simulink model "AC_motor"  (R2025b)
settings: Solver=VariableStepAuto  StartTime=0.0  StopTime=10  RelTol=1e-3
libraries: nesl_utility x11, ee_lib x10, fl_lib x8
settings Model: Creator=Администратор  LastModifiedBy=Администратор

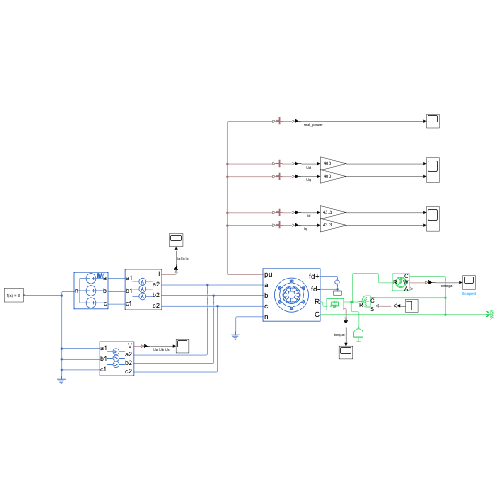
[thumbnail: Simulink's stored preview of the top-level diagram]
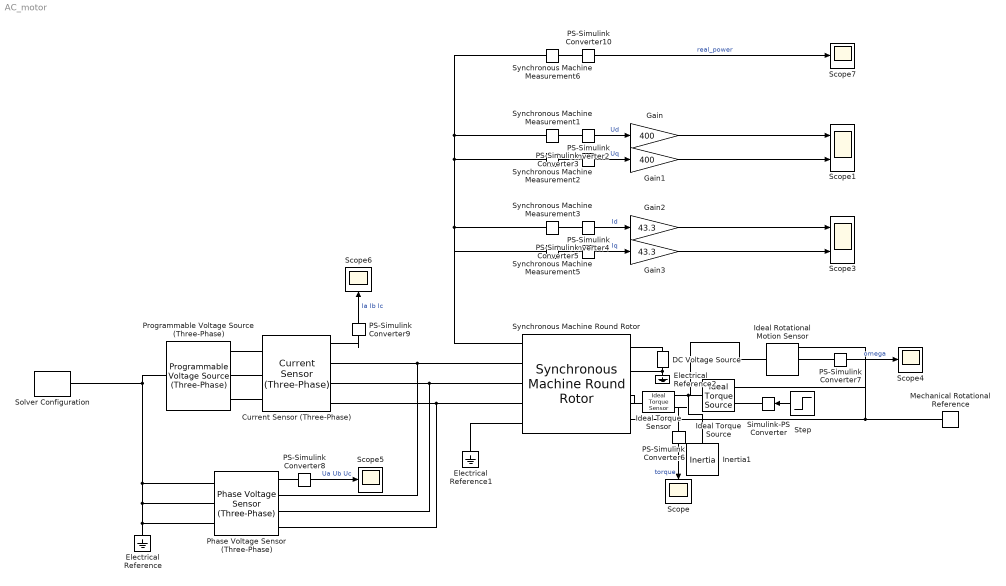
== system AC_motor ==
  Current Sensor (Three-Phase) : ee_lib/Sensors & Transducers/Current Sensor (Three-Phase)
      settings: InternalSimscapePortConfiguration="{\"Bottom\":[],\"Left\":[{\"id\":\"a1\",\"label\":\"a1\",\"type\":\"foundation.electrical.electrical\"},{\"id\":\"b1\",\"label\":\"b1\",\"type\":\"foundation.electrical.electrical\"},{\"id\":\"c1\",\"label\":\"c1\",\"type\":\"foundation.electrical.electrical\"}],\"Right\":[{\"id\":\"I_output\",\"label\":\"I\",\"type\":\"output\"},{\"id\":\"a2\",\"label\":\"a2\",\"type\":\"foundation.electrical.electrical\"},{\"id\":\"b2\",\"label\":\"b2\",\"type\":\"foundation.electrical.electrical\"},{\"id\":\"c2\",\"label\":\"c2\",\"type\":\"foundation.electrical.electrical\"}],\"Top\":[]}"
  DC Voltage Source : ee_lib/Additional Components/SPICE Sources/DC Voltage Source  DC=24 V
  Electrical Reference : fl_lib/Electrical/Electrical Elements/Electrical Reference
  Electrical Reference1 : fl_lib/Electrical/Electrical Elements/Electrical Reference
  Electrical Reference2 : fl_lib/Electrical/Electrical Elements/Electrical Reference
  Gain : Gain  Gain=400
  Gain1 : Gain  Gain=400
  Gain2 : Gain  Gain=43.3
  Gain3 : Gain  Gain=43.3
  Ideal Rotational Motion Sensor : fl_lib/Mechanical/Mechanical Sensors/Ideal Rotational Motion Sensor  reference=foundation.enum.MeasurementReference.difference  acceleration_port=false  velocity_port=true  position_port=true  wrap_angle=false  offset=0 rad
  Ideal Torque Sensor : fl_lib/Mechanical/Mechanical Sensors/Ideal Torque Sensor
  Ideal Torque Source : fl_lib/Mechanical/Mechanical Sources/Ideal Torque Source
  Inertia1 : fl_lib/Mechanical/Rotational Elements/Inertia  inertia=0.05 kg*m^2  num_ports=foundation.enum.numPorts2.one  w_specify=off  w_priority=High  w=0 rad/s  w_nominal_specify=off  w_nominal_value=1  w_nominal_unit=rad/s  t_specify=off  t_priority=None  t=0 N*m  t_nominal_specify=off  t_nominal_value=1  t_nominal_unit=N*m
  Mechanical Rotational Reference : fl_lib/Mechanical/Rotational Elements/Mechanical Rotational Reference
  PS-Simulink Converter{2..10} (9 alike) : nesl_utility/PS-Simulink Converter  PhysicalDomain=network_engine_domain  SubClassName=ps_output  LeftPortType=input  RightPortType=output  PseudoPeriodic=off  Frequencies=[]  VectorFormat=inherit  Unit=inherit  AffineConversion=off
  Phase Voltage Sensor (Three-Phase) : ee_lib/Sensors & Transducers/Phase Voltage Sensor (Three-Phase)
      settings: InternalSimscapePortConfiguration="{\"Bottom\":[],\"Left\":[{\"id\":\"a1\",\"label\":\"a1\",\"type\":\"foundation.electrical.electrical\"},{\"id\":\"b1\",\"label\":\"b1\",\"type\":\"foundation.electrical.electrical\"},{\"id\":\"c1\",\"label\":\"c1\",\"type\":\"foundation.electrical.electrical\"}],\"Right\":[{\"id\":\"V_output\",\"label\":\"V\",\"type\":\"output\"},{\"id\":\"a2\",\"label\":\"a2\",\"type\":\"foundation.electrical.electrical\"},{\"id\":\"b2\",\"label\":\"b2\",\"type\":\"foundation.electrical.electrical\"},{\"id\":\"c2\",\"label\":\"c2\",\"type\":\"foundation.electrical.electrical\"}],\"Top\":[]}"
  Programmable Voltage Source (Three-Phase) : ee_lib/Sources/Programmable Voltage Source (Three-Phase)  magnitude_type=ee.enum.timechanging.constant  vline_rms=400 V  magn_ramp=1 V/s  magn_step=1 V  magn_modu_magn=1 V  magn_modu_freq=1 Hz  magn_t1=1 s  magn_t2=2 s  frequency_type=ee.enum.timechanging.constant  freq=50 Hz  freq_ramp=1 Hz/s  freq_step=1 Hz  freq_modu_magn=1 Hz  freq_modu_freq=1 Hz  freq_t1=1 s  freq_t2=2 s  phase_type=ee.enum.timechanging.constant  shift=0 deg  phase_ramp=1 deg/s  phase_step=1 deg  phase_modu_magn=1 deg  phase_modu_freq=1 Hz  phase_t1=1 s  phase_t2=2 s  impedance_option=1  SShortCircuit=1e6 A*V  XR=15  R=0.01 Ohm  L=3.97e-4 H  G_parasitic=1e-6 1/Ohm  harmonic_option=0  harmonic_orders=[5, 7, 11, 13]  harmonic_ratios=[.1, .1, .1, .1]  harmonic_shifts=[0, 0, 0, 0] deg  harmonic_sequences=[1, 1, 1, 1]  harmonic_t1=-inf s  harmonic_t2=inf s  I_specify=off  I_priority=None  I=[0, 0, 0] A  I_nominal_specify=off  I_nominal_value=1  I_nominal_unit=A  V_specify=off  V_priority=None  V=[0, 0, 0] V  V_nominal_specify=off  V_nominal_value=1  V_nominal_unit=V
      settings: InternalSimscapePortConfiguration="{\"Bottom\":[],\"Left\":[{\"id\":\"n\",\"label\":\"n\",\"type\":\"foundation.electrical.electrical\"}],\"Right\":[{\"id\":\"a\",\"label\":\"a\",\"type\":\"foundation.electrical.electrical\"},{\"id\":\"b\",\"label\":\"b\",\"type\":\"foundation.electrical.electrical\"},{\"id\":\"c\",\"label\":\"c\",\"type\":\"foundation.electrical.electrical\"}],\"Top\":[]}"
  Scope{,4..7} (5 alike) : Scope
      Scope settings: ActiveDisplayYMinimum=-180.7119358740091  ActiveDisplayYMaximum=164.56605667800315  DataLoggingVariableName=ScopeData3
      Scope4 settings: ActiveDisplayYMinimum=121.85410021778432  ActiveDisplayYMaximum=208.87010775351609  DataLoggingVariableName=ScopeData4
      Scope5 settings: ActiveDisplayYMinimum=-4339.2016290441516  ActiveDisplayYMaximum=1807.2818447656446  DataLoggingVariableName=ScopeData5
      Scope6 settings: ActiveDisplayYMinimum=-436.89999743649622  ActiveDisplayYMaximum=142.21320753429535  DataLoggingVariableName=ScopeData6
      Scope7 settings: ActiveDisplayYMinimum=-0.70641268155042636  ActiveDisplayYMaximum=-0.5696896154734612  DataLoggingVariableName=ScopeData7
  Scope1 : Scope  NumInputPorts=2
      settings: ActiveDisplayYMinimum=-0.68803937842332719  ActiveDisplayYMaximum=0.70916847198511146
  Scope3 : Scope  NumInputPorts=2
      settings: ActiveDisplayYMinimum=-1.0232590834035449  ActiveDisplayYMaximum=0.66835925847558086
  Simulink-PS Converter : nesl_utility/Simulink-PS Converter  PhysicalDomain=network_engine_domain  SubClassName=ps_input  LeftPortType=input  RightPortType=output  PseudoPeriodic=off  Frequencies=[]  NoiseDistribution=none  NoiseParameters=[]  Unit=1  AffineConversion=off  FilteringAndDerivatives=provide  SimscapeFilterOrder=1  InputFilterTimeConstant=0.001  UdotUserProvided=0
  Solver Configuration : nesl_utility/Solver Configuration  PhysicalDomain=network_engine_domain  SubClassName=solver  LeftPortType=input  RightPortType=generic  Tones=[]  Harmonics=[]  SimulateNoise=off  Profile=off  UseLocalSampling=off  EnableSwitchedLinearOptims=on  FrequencyDomain=off  UseCCode=off  RelTol=0.001  AbsTol=0.001  MinStep=1e-09  ToWorkspace=off  RevertToSquareIcSolve=off  NumHomotopyIterations=100  PhasorMode=off  PhasorModeNumHarmonics=1  ConsistencySolver=NEWTON_XTOL_AFTER_FTOL  IndexReductionMethod=DerivativeReplacement  DoDC=off  ResidualTolerance=1e-09  ConsistencyTolSource=GLOBAL  ConsistencyAbsTol=0.001  ConsistencyRelTol=0.001  ConsistencyTolFactor=0.001  UseLocalSolver=off  LocalSolverChoice=NE_BACKWARD_EULER_ADVANCER  ResolveIndetEquations=on  FunctionEvalNumThread=1  LocalSolverSampleTime=0.001  DoFixedCost=off  MaxNonlinIter=3  MaxModeIter=2  ComputeImpulses=off  ImpulseIterations=2  LinearAlgebra=auto  LinearAlgebraNumThread=0  EquationFormulation=NE_TIME_EF  DelaysMemoryBudget=1024  AutomaticFiltering=on  FilteringTimeConstant=0.001  PartitionStorageMethod=AS_NEEDED  PartitionMemoryBudget=1024  PartitionMethod=ROBUST  MultibodyUseLocalSolver=off  MultibodyLocalSolverChoice=ODE1  MultibodyLocalSolverSampleTime=0.001
  Step : Step  Time=5  After=-100  SampleTime=0
  Synchronous Machine Measurement1 : ee_lib/Electromechanical/Synchronous/Synchronous Machine Measurement  output_idx=5
      settings: InternalSimscapePortConfiguration="{\"Bottom\":[],\"Left\":[{\"id\":\"pu_input\",\"label\":\"pu\",\"type\":\"input\"}],\"Right\":[{\"id\":\"pu_output\",\"label\":\"o\",\"type\":\"output\"}],\"Top\":[]}"
  Synchronous Machine Measurement2 : ee_lib/Electromechanical/Synchronous/Synchronous Machine Measurement  output_idx=6
      settings: InternalSimscapePortConfiguration="{\"Bottom\":[],\"Left\":[{\"id\":\"pu_input\",\"label\":\"pu\",\"type\":\"input\"}],\"Right\":[{\"id\":\"pu_output\",\"label\":\"o\",\"type\":\"output\"}],\"Top\":[]}"
  Synchronous Machine Measurement3 : ee_lib/Electromechanical/Synchronous/Synchronous Machine Measurement  output_idx=8
      settings: InternalSimscapePortConfiguration="{\"Bottom\":[],\"Left\":[{\"id\":\"pu_input\",\"label\":\"pu\",\"type\":\"input\"}],\"Right\":[{\"id\":\"pu_output\",\"label\":\"o\",\"type\":\"output\"}],\"Top\":[]}"
  Synchronous Machine Measurement5 : ee_lib/Electromechanical/Synchronous/Synchronous Machine Measurement  output_idx=9
      settings: InternalSimscapePortConfiguration="{\"Bottom\":[],\"Left\":[{\"id\":\"pu_input\",\"label\":\"pu\",\"type\":\"input\"}],\"Right\":[{\"id\":\"pu_output\",\"label\":\"o\",\"type\":\"output\"}],\"Top\":[]}"
  Synchronous Machine Measurement6 : ee_lib/Electromechanical/Synchronous/Synchronous Machine Measurement  output_idx=12
      settings: InternalSimscapePortConfiguration="{\"Bottom\":[],\"Left\":[{\"id\":\"pu_input\",\"label\":\"pu\",\"type\":\"input\"}],\"Right\":[{\"id\":\"pu_output\",\"label\":\"o\",\"type\":\"output\"}],\"Top\":[]}"
  Synchronous Machine Round Rotor : ee_lib/Electromechanical/Synchronous/Synchronous Machine Round Rotor  port_option=ee.enum.threePhasePort.expanded  SRated=30e3 A*V  VRated=400 V  FRated=50 Hz  nPolePairs=2  param_option=ee.enum.sm.parameterization.fundamental  fieldCircuitParameterization_option=ee.enum.sm.fieldparameterization.voltage  baseEfd=24 V  baseIfd=1300 A  zero_sequence=ee.enum.park.zerosequence.include  axes_param=ee.enum.rotorangle.daxis  Ladu=0.03  Laqu=0.03  L0=0.005  Ll=0.005  Ra=0.1  Lfd=0.05  Rfd=2  L1d=0.01  R1d=1  L1q=0.01  R1q=1  L2q=0.005  R2q=1  Xl=0.15  Xd=1.81  Xq=1.76  X0=0.15  Xdd=0.3  Xqd=0.65  Xddd=0.23  Xqdd=0.25  d_option=ee.enum.circuit.open  Td0d=8 s  Tdd=1.3260 s  Td0dd=0.03 s  Tddd=0.0230 s  q_option=ee.enum.circuit.open  Tq0d=1 s  Tqd=0.3693 s  Tq0dd=0.07 s  Tqdd=0.0269 s  saturation_option=ee.enum.saturation.exclude  saturation_ifd=[0, .48, .76, 1.38, 1.79]  saturation_Vag=[0, .8, 1.08, 1.31, 1.4]  initialization_option=ee.enum.sm.initialization.mechanical  source_type=ee.enum.sm.load_flow_source_type.Swing  Vmag0=24e3 V  Vang0=0 deg  Pt0=500e6 A*V  Qt0=0 A*V  minimum_pu=0.95  phase_search_range=[-inf, inf] deg  gmin=1e-6 S  connection_option=ee.enum.Connection.wye  num_q_dampers=2  rotor_offset=-pi / 2 rad  pu_psid_specify=off  pu_psid_priority=None  pu_psid=0  pu_psid_nominal_specify=off  pu_psid_nominal_value=1  pu_psid_nominal_unit=1  pu_psiq_specify=off  pu_psiq_priority=None  pu_psiq=0  pu_psiq_nominal_specify=off  pu_psiq_nominal_value=1  pu_psiq_nominal_unit=1  pu_psifd_specify=off  pu_psifd_priority=None  pu_psifd=0  pu_psifd_nominal_specify=off  pu_psifd_nominal_value=1  pu_psifd_nominal_unit=1  pu_psi1d_specify=off  pu_psi1d_priority=None  pu_psi1d=0  pu_psi1d_nominal_specify=off  pu_psi1d_nominal_value=1  pu_psi1d_nominal_unit=1  pu_psi1q_specify=off  pu_psi1q_priority=None  pu_psi1q=0  pu_psi1q_nominal_specify=off  pu_psi1q_nominal_value=1  pu_psi1q_nominal_unit=1  pu_psi2q_specify=off  pu_psi2q_priority=None  pu_psi2q=0  pu_psi2q_nominal_specify=off  pu_psi2q_nominal_value=1  pu_psi2q_nominal_unit=1  angular_position_diff_specify=off  angular_position_diff_priority=None  angular_position_diff=180 deg  angular_position_diff_nominal_specify=off  angular_position_diff_nominal_value=1  angular_position_diff_nominal_unit=deg  Tmeas=298.15 K  alpha=3.93e-3 1/K  stator_thermal_mass=100 J/K  rotor_thermal_mass=200 J/K  temperatureA_specify=off  temperatureA_priority=High  temperatureA=25 degC  temperatureA_nominal_specify=off  temperatureA_nominal_value=1  temperatureA_nominal_unit=degC  temperatureB_specify=off  temperatureB_priority=High  temperatureB=25 degC  temperatureB_nominal_specify=off  temperatureB_nominal_value=1  temperatureB_nominal_unit=degC  temperatureC_specify=off  temperatureC_priority=High  temperatureC=25 degC  temperatureC_nominal_specify=off  temperatureC_nominal_value=1  temperatureC_nominal_unit=degC  temperatureR_specify=off  temperatureR_priority=High  temperatureR=25 degC  temperatureR_nominal_specify=off  temperatureR_nominal_value=1  temperatureR_nominal_unit=degC
      settings: InternalSimscapePortConfiguration="{\"Bottom\":[],\"Left\":[{\"id\":\"fd_p\",\"label\":\"fd+\",\"type\":\"foundation.electrical.electrical\"},{\"id\":\"fd_n\",\"label\":\"fd-\",\"type\":\"foundation.electrical.electrical\"},{\"id\":\"R\",\"label\":\"R\",\"type\":\"foundation.mechanical.rotational.rotational\"},{\"id\":\"C\",\"label\":\"C\",\"type\":\"foundation.mechanical.rotational.rotational\"}],\"Right\":[{\"id\":\"pu_output\",\"label\":\"pu\",\"type\":\"output\"},{\"id\":\"a\",\"label\":\"a\",\"type\":\"foundation.electrical.electrical\"},{\"id\":\"b\",\"label\":\"b\",\"type\":\"foundation.electrical.electrical\"},{\"id\":\"c\",\"label\":\"c\",\"type\":\"foundation.electrical.electrical\"},{\"id\":\"n\",\"label\":\"n\",\"type\":\"foundation.electrical.electrical\"}],\"Top\":[]}"
  wires:
  PS-Simulink Converter2/1 -> Gain/1  "Ud"
  PS-Simulink Converter3/1 -> Gain1/1  "Uq"
  PS-Simulink Converter4/1 -> Gain2/1  "Id"
  PS-Simulink Converter5/1 -> Gain3/1  "Iq"
  PS-Simulink Converter6/1 -> Scope/1  "torque"
  Step/1 -> Simulink-PS Converter/1
  PS-Simulink Converter7/1 -> Scope4/1  "omega"
  PS-Simulink Converter8/1 -> Scope5/1  "Ua Ub Uc"
  PS-Simulink Converter9/1 -> Scope6/1  "Ia Ib Ic"
  Gain/1 -> Scope1/1
  Gain1/1 -> Scope1/2
  Gain3/1 -> Scope3/2
  Gain2/1 -> Scope3/1
  PS-Simulink Converter10/1 -> Scope7/1  "real_power"
  connections:
  Synchronous Machine Round Rotor/LConn1 -- DC Voltage Source/LConn1
  Phase Voltage Sensor (Three-Phase)/RConn3 -- Current Sensor (Three-Phase)/RConn3 -- Synchronous Machine Round Rotor/RConn3
  Phase Voltage Sensor (Three-Phase)/RConn4 -- Current Sensor (Three-Phase)/RConn4 -- Synchronous Machine Round Rotor/RConn4
  Phase Voltage Sensor (Three-Phase)/RConn2 -- Current Sensor (Three-Phase)/RConn2 -- Synchronous Machine Round Rotor/RConn2
  Electrical Reference/LConn1 -- Phase Voltage Sensor (Three-Phase)/LConn3 -- Phase Voltage Sensor (Three-Phase)/LConn2 -- Phase Voltage Sensor (Three-Phase)/LConn1 -- Solver Configuration/RConn1 -- Programmable Voltage Source (Three-Phase)/LConn1
  Synchronous Machine Round Rotor/RConn5 -- Electrical Reference1/LConn1
  DC Voltage Source/RConn1 -- Electrical Reference2/LConn1 -- Synchronous Machine Round Rotor/LConn2
  Mechanical Rotational Reference/LConn1 -- Synchronous Machine Round Rotor/LConn4 -- Ideal Rotational Motion Sensor/RConn1 -- Ideal Torque Source/RConn2
  Simulink-PS Converter/RConn1 -- Ideal Torque Source/RConn1
  Synchronous Machine Measurement1/LConn1 -- Synchronous Machine Measurement6/LConn1 -- Synchronous Machine Measurement2/LConn1 -- Synchronous Machine Measurement3/LConn1 -- Synchronous Machine Measurement5/LConn1 -- Synchronous Machine Round Rotor/RConn1
  PS-Simulink Converter4/LConn1 -- Synchronous Machine Measurement3/RConn1
  PS-Simulink Converter3/LConn1 -- Synchronous Machine Measurement2/RConn1
  PS-Simulink Converter2/LConn1 -- Synchronous Machine Measurement1/RConn1
  PS-Simulink Converter5/LConn1 -- Synchronous Machine Measurement5/RConn1
  Inertia1/LConn1 -- Ideal Rotational Motion Sensor/LConn1 -- Ideal Torque Source/LConn1 -- Ideal Torque Sensor/RConn1
  Ideal Torque Sensor/LConn1 -- Synchronous Machine Round Rotor/LConn3
  Ideal Torque Sensor/RConn2 -- PS-Simulink Converter6/LConn1
  PS-Simulink Converter7/LConn1 -- Ideal Rotational Motion Sensor/RConn2
  Phase Voltage Sensor (Three-Phase)/RConn1 -- PS-Simulink Converter8/LConn1
  Current Sensor (Three-Phase)/LConn1 -- Programmable Voltage Source (Three-Phase)/RConn1
  Current Sensor (Three-Phase)/LConn2 -- Programmable Voltage Source (Three-Phase)/RConn2
  Programmable Voltage Source (Three-Phase)/RConn3 -- Current Sensor (Three-Phase)/LConn3
  PS-Simulink Converter9/LConn1 -- Current Sensor (Three-Phase)/RConn1
  PS-Simulink Converter10/LConn1 -- Synchronous Machine Measurement6/RConn1
